simulink model "s0211d"  (Simulink 6.0)
settings: Solver=ode45  StartTime=0.0  StopTime=1  MaxStep=0.02  RelTol=1e-3
values from neighbouring files (symbols this model uses):
  C = C*1e-6    (= 0.0001)    [m0203.m]    (also in m0204.m; m0205.m; m0207.m; m0211d.m)
  R = R*1e3    (= 1000)    [m0203.m]    (also in m0204.m; m0205.m; m0207.m; m0211d.m = 2000)
settings Model: LastModifiedBy=Froriep

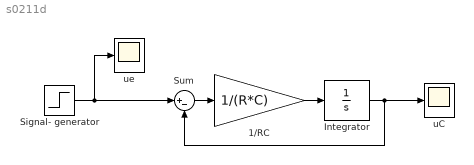
== system s0211d ==
  1/RC : Gain  Gain=1/(R*C)
  Integrator : Integrator
  Signal- generator : Step  Time=.2  SampleTime=0
  Sum : Sum  Inputs=|+-
  uC : Scope
      settings: YMin=-0.2  YMax=1.2
  ue : Scope
      settings: YMin=-0.2  YMax=1.2
  wires:
  Sum/1 -> 1/RC/1
  1/RC/1 -> Integrator/1
  Integrator/1 -> Sum/2, uC/1
  Signal- generator/1 -> Sum/1, ue/1
